simulink model "traffic_light_system_using_Arduino_and_LEDs"  (R2022b)
settings: Solver=FixedStepDiscrete  StartTime=0.0  StopTime=inf  RelTol=1e-3  EnableMultiTasking=on
libraries: simulink x6, arduinolib x3
settings Model: ExtModeTrigDuration=2  Creator=ahmed  LastModifiedBy=ahmed
settings OptimizationCC: EnhancedBackFolding=on  PassReuseOutputArgsAs=Individual arguments  ZeroExternalMemoryAtStartup=off  ZeroInternalMemoryAtStartup=off  MaxStackSize=64  OptimizeBlockOrder=speed  DifferentSizesBufferReuse=on  OptimizationCustomize=off  EfficientTunableParamExpr=on
settings DebuggingCC: ParameterTunabilityLossMsg=error
settings HardwareCC: ProdBitPerInt=16  ProdBitPerPointer=16  ProdBitPerSizeT=16  ProdBitPerPtrDiffT=16  ProdLargestAtomicFloat=None  ProdWordSize=8  ProdHWDeviceType=Atmel->AVR
settings SFSimCC: MATLABDynamicMemAlloc=off
settings RTWCC: Description=Embedded Coder  SystemTargetFile=ert.tlc  HardwareBoard=Arduino Uno  TLCOptions=-aInlineSetEventsForThisBaseRateFcn=TLC_FALSE -aSuppressMultiTaskScheduler=TLC_FALSE -aRateBasedStepFcn=1  TemplateMakefile=ert_default_tmf  Toolchain=Arduino AVR  BuildConfiguration=Faster Runs
settings CodeAppCC: ForceParamTrailComments=on  IgnoreCustomStorageClasses=off  OperatorAnnotations=on  SimulinkDataObjDesc=on  SFDataObjDesc=on  InsertBlockDesc=on
settings ERTTargetCC: SupportContinuousTime=on  SupportVariableSizeSignals=on  ExtModeTransport=3  ExtModeStaticAlloc=on  ExtModeAutomaticAllocSize=off  ExtModeStaticAllocSize=250  ExtModeMexFile=ext_xcp  ExtModeIntrfLevel=Level2 - Open

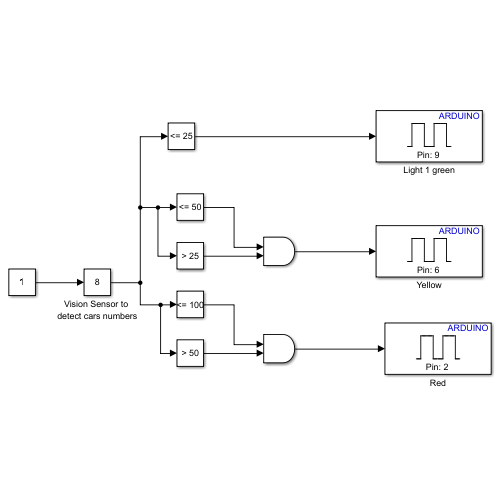
[thumbnail: Simulink's stored preview of the top-level diagram]
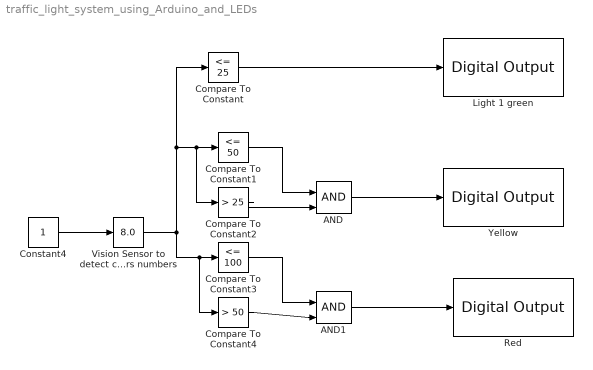
== system traffic_light_system_using_Arduino_and_LEDs ==
  AND : Logic  IconShape=distinctive  AllPortsSameDT=off  OutDataTypeStr=boolean
  AND1 : Logic  IconShape=distinctive  AllPortsSameDT=off  OutDataTypeStr=boolean
  Compare To Constant : simulink/Logic and Bit Operations/Compare To Constant  relop=<=  const=25  OutDataTypeStr=boolean
  Compare To Constant1 : simulink/Logic and Bit Operations/Compare To Constant  relop=<=  const=50  OutDataTypeStr=boolean
  Compare To Constant2 : simulink/Logic and Bit Operations/Compare To Constant  relop=>  const=25  OutDataTypeStr=boolean
  Compare To Constant3 : simulink/Logic and Bit Operations/Compare To Constant  relop=<=  const=100  OutDataTypeStr=boolean
  Compare To Constant4 : simulink/Logic and Bit Operations/Compare To Constant  relop=>  const=50  OutDataTypeStr=boolean
  Constant4 : Constant
  Light 1 green : arduinolib/Digital Output  pinNumber=9  Direction=output  blockPlatform=arduino
  Red : arduinolib/Digital Output  pinNumber=2  Direction=output  blockPlatform=arduino
  Vision Sensor to detect cars numbers : simulink/Math Operations/Slider Gain  gain=8.0  low=0  high=100
  Yellow : arduinolib/Digital Output  pinNumber=6  Direction=output  blockPlatform=arduino
  wires:
  Constant4/1 -> Vision Sensor to detect cars numbers/1
  Vision Sensor to detect cars numbers/1 -> Compare To Constant2/1, Compare To Constant1/1, Compare To Constant/1, Compare To Constant4/1, Compare To Constant3/1
  Compare To Constant2/1 -> AND/2
  Compare To Constant1/1 -> AND/1
  Compare To Constant3/1 -> AND1/1
  Compare To Constant4/1 -> AND1/2
  Compare To Constant/1 -> Light 1 green/1
  AND/1 -> Yellow/1
  AND1/1 -> Red/1
